simulink model "Motor_model"  (R2016b)
settings: Solver=VariableStepAuto  StartTime=0.0  StopTime=5  MaxStep=0.01  RelTol=1e-3
libraries: simulink x1
settings Model: Creator=Administrator  LastModifiedBy=Administrator

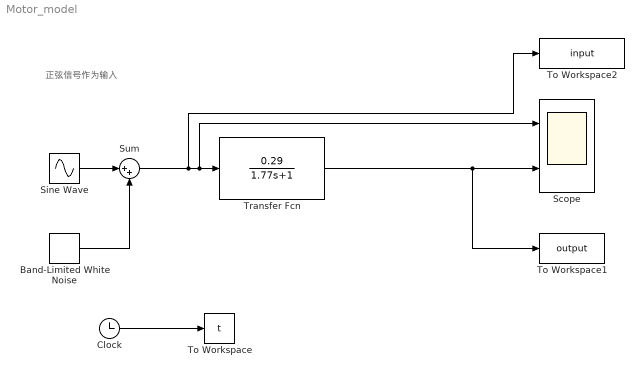
== system Motor_model ==
  note: 正弦信号作为输入
  Band-Limited White Noise : simulink/Sources/Band-Limited White Noise  Cov=[0.0001]  Ts=0.01  seed=[23341]
  Clock : Clock
  Scope : Scope  NumInputPorts=2
  Sine Wave : Sin  Frequency=3  SampleTime=0
  Sum : Sum  Inputs=|++
  To Workspace : ToWorkspace  VariableName=t  SampleTime=-1
  To Workspace1 : ToWorkspace  VariableName=output  SampleTime=-1
  To Workspace2 : ToWorkspace  VariableName=input  SampleTime=-1
  Transfer Fcn : TransferFcn  Numerator=[0.29]  Denominator=[1.77 1]
  wires:
  Transfer Fcn/1 -> To Workspace1/1, Scope/2
  Clock/1 -> To Workspace/1
  Sine Wave/1 -> Sum/1
  Sum/1 -> To Workspace2/1, Scope/1, Transfer Fcn/1
  Band-Limited White Noise/1 -> Sum/2
